simulink model "hopeForSarah"  (R2019a)
settings: Solver=ode1  StartTime=0.0  StopTime=2.5  FixedStep=Ts_Power  RelTol=1e-3
PostLoadFcn:
  | %% Init for wind PnO models - global system parameters
  | OVERRIDE_SSN_MEMORY_LIMIT=1;
  | Ts=50e-6;
  | % Ts=50e-10;
  | Ts_Power=Ts;
  | Ts_Control=2*Ts;
  | freq = 50;
  | Fnom=freq;
  | Vac=400e3;
InitFcn:
  | %% Init for wind PnO models - global system parameters
  | OVERRIDE_SSN_MEMORY_LIMIT=1;
  | Ts=50e-6;
  | % Ts=50e-10;
  | Ts_Power=Ts;
  | Ts_Control=2*Ts;
  | freq = 50;
  | Fnom=freq;
  | Vac=225e3;
values from neighbouring files (symbols this model uses):
  sub_posCap = 0.16e-006    (= 1.6e-07)    [variable.m]
  sub_posInd = 0.001400563    [variable.m]
  sub_posR = 0.036    [variable.m]
  sub_zeroCap = 0.053333e-006    (= 5.3333e-08)    [variable.m]
  sub_zeroInd = 0.00420169    [variable.m]
  sub_zeroR = 0.108    [variable.m]
  transfo_L1 = 0.05999374    [variable.m]
  transfo_L2 = 0.05999374    [variable.m]
  transfo_R1 = 0.000866667    [variable.m]
  transfo_R2 = 0.00086667    [variable.m]
undefined symbols (not defined in the file or in its folder): D1, D11, Delta, den, DiscIntNeverNeededParam, dx, find_system, gcbh, num, out_Buses, out_WindFarms, sps_rtmsupport
libraries: powerlib x284, simulink x144, powerlib_meascontrol x144, eeSinusoidalMeasurement x74, elements x52, spsVIMeasurementModel x48, simulink_extras x48, eePowerMeasurement x23
(part 3 of 30)

== system hopeForSarah/SC_Console/Subsystem ==
  In1 : Inport
  Bus Selector : BusSelector  OutputSignals=Vabc_grid (pu),Iabc_conv (pu),P_grid,Q_grid
  Bus Selector1 : BusSelector  OutputSignals=Q_grid (y: nom; b: measured),V_dc (y: nom; b: measured),I_abc (A),id,iq,theta_PLL
  Bus Selector2 : BusSelector  OutputSignals=Idc_gen+grid,I_cap+chopper,Pgrid,vdc
  Bus Selector3 : BusSelector  OutputSignals=Vabc (kV),Iabc,PQ,Pelec (MW)
  Bus Selector4 : BusSelector  OutputSignals=Vabc_pu_mag,Iabc_pu_mag,PQ,Pelec_pu
  Bus Selector5 : BusSelector  OutputSignals=WindTurbine_GridSide,WindTurbine_ConverterSide,WindTurbine_DCSide,WindTurbine_PhasetoGroundMeasurements,WindTurbine_puMeasurements,Windturbine_FaultvsGridFRTRequirements,WindTurbine_Displays
  Bus Selector6 : BusSelector  OutputSignals=Vabc pu mag,Grid Code FRT requirements
  Bus Selector7 : BusSelector  OutputSignals=Disconnection_Trigger,Time under FRT,Minimum Voltage pu,Peak POC Current pu,FRT Disconnection Time
  Bus Selector8 : BusSelector  OutputSignals=P_pu,Q_pu
  Bus Selector9 : BusSelector  OutputSignals=P (MW),Q (MVA)
  Goto14 : Goto  Commented=on  GotoTag=Pgrid  TagVisibility=global
  Goto20 : Goto  Commented=on  GotoTag=Vabc_pu_mag  TagVisibility=global
  Mux : Mux  Inputs=2
  Mux1 : Mux  Inputs=2
  tag scope: Disconnection_trigger=global, FRT_disconnection_time=global, FRT_grid_code_requirements=global, FRT_time=global, I_capANDchopper=global, Iabc=global, Iabc_conv_pu=global, Iabc_pu_mag=global, Iabc_ref=global, Idc_genANDgrid=global, Minimum_Voltage_pu=global, PQ=global, PQ_pu=global, Peak_POC_current_pu=global, Pelec=global, Pelec_pu=global, Pgrid=global, Qgrid=global, Qgrid_nomandmeas=global, Theta_PLL=global, Vabc_grid_pu=global, Vabc_kV=global, Vabc_pu_mag=global, Vdc=global, Vdc_nomandmeas=global, id=global, iq=global
  wires:
  In1/1 -> Bus Selector5/1
  Bus Selector5/1 -> Bus Selector/1  "<WindTurbine_GridSide>"
  Bus Selector5/2 -> Bus Selector1/1  "<WindTurbine_ConverterSide>"
  Bus Selector5/3 -> Bus Selector2/1  "<WindTurbine_DCSide>"
  Bus Selector5/4 -> Bus Selector3/1  "<WindTurbine_PhasetoGroundMeasurements>"
  Bus Selector5/5 -> Bus Selector4/1  "<WindTurbine_puMeasurements>"
  Bus Selector5/6 -> Bus Selector6/1  "<Windturbine_FaultvsGridFRTRequirements>"
  Bus Selector5/7 -> Bus Selector7/1  "<WindTurbine_Displays>"
  Bus Selector/1 -> [Vabc_grid_pu]  "<Vabc_grid (pu)>"
  Bus Selector/2 -> [Iabc_conv_pu]  "<Iabc_conv (pu)>"
  Bus Selector/3 -> [Pgrid]  "<P_grid>"
  Bus Selector/4 -> [Qgrid]  "<Q_grid>"
  Bus Selector1/1 -> [Qgrid_nomandmeas]  "<Q_grid (y: nom; b: measured)>"
  Bus Selector1/2 -> [Vdc_nomandmeas]  "<V_dc (y: nom; b: measured)>"
  Bus Selector1/3 -> [Iabc_ref]  "<I_abc (A)>"
  Bus Selector1/4 -> [id]  "<id>"
  Bus Selector1/5 -> [iq]  "<iq>"
  Bus Selector1/6 -> [Theta_PLL]  "<theta_PLL>"
  Bus Selector2/1 -> [Idc_genANDgrid]  "<Idc_gen+grid>"
  Bus Selector2/2 -> [I_capANDchopper]  "<I_cap+chopper>"
  Bus Selector2/3 -> Goto14/1  "<Pgrid>"
  Bus Selector2/4 -> [Vdc]  "<vdc>"
  Bus Selector3/1 -> [Vabc_kV]  "<Vabc (kV)>"
  Bus Selector3/2 -> [Iabc]  "<Iabc>"
  Bus Selector3/4 -> [Pelec]  "<Pelec (MW)>"
  Bus Selector4/1 -> [Vabc_pu_mag]  "<Vabc_pu_mag>"
  Bus Selector4/2 -> [Iabc_pu_mag]  "<Iabc_pu_mag>"
  Bus Selector4/3 -> Bus Selector8/1  "<PQ>"
  Bus Selector4/4 -> [Pelec_pu]  "<Pelec_pu>"
  Bus Selector6/1 -> Goto20/1  "<Vabc pu mag>"
  Bus Selector6/2 -> [FRT_grid_code_requirements]  "<Grid Code FRT requirements>"
  Bus Selector7/1 -> [Disconnection_trigger]  "<Disconnection_Trigger>"
  Bus Selector7/2 -> [FRT_time]  "<Time under FRT>"
  Bus Selector7/3 -> [Minimum_Voltage_pu]  "<Minimum Voltage pu>"
  Bus Selector7/4 -> [Peak_POC_current_pu]  "<Peak POC Current pu>"
  Bus Selector7/5 -> [FRT_disconnection_time]  "<FRT Disconnection Time>"
  Bus Selector8/1 -> Mux/1  "<P_pu>"
  Bus Selector8/2 -> Mux/2  "<Q_pu>"
  Mux/1 -> [PQ_pu]  "PQ (1:P_pu;2:Q_pu)"
  Mux1/1 -> [PQ]  "PQ (1:P;2:Q)"
  Bus Selector9/2 -> Mux1/2  "<Q (MVA)>"
  Bus Selector9/1 -> Mux1/1  "<P (MW)>"
  Bus Selector3/3 -> Bus Selector9/1  "<PQ>"

== system hopeForSarah/SC_Console/Subsystem1 ==
  In1 : Inport
  Bus Selector1 : BusSelector  OutputSignals=Vabc,Iabc,V mag,I mag,PQ
  tag scope: Bus_Iabc=global, Bus_Imag=global, Bus_PQ=global, Bus_Vabc=global, Bus_Vmag=global
  wires:
  In1/1 -> Bus Selector1/1
  Bus Selector1/1 -> [Bus_Vabc]  "<Vabc>"
  Bus Selector1/2 -> [Bus_Iabc]  "<Iabc>"
  Bus Selector1/5 -> [Bus_PQ]  "<PQ>"
  Bus Selector1/4 -> [Bus_Imag]  "<I mag>"
  Bus Selector1/3 -> [Bus_Vmag]  "<V mag>"

== system hopeForSarah/SC_Console/Subsystem3 ==
  Disconnection_Trigger : Inport
  String Constant1 : StringConstant  String="\"FRT limit surpassed\""
  String Constant2 : StringConstant  String="\"\""
  Switch1 : Switch  Criteria=u2 > Threshold
  Disconnection message : Outport  VectorParamsAs1DForOutWhenUnconnected=on
  wires:
  String Constant1/1 -> Switch1/1
  Switch1/1 -> Disconnection message/1  "Disconnection message"
  Disconnection_Trigger/1 -> Switch1/2
  String Constant2/1 -> Switch1/3

== system hopeForSarah/SC_Console/Subsystem4 ==
  Fault Current abc : Inport
  From A to kA : Gain  Gain=1/1000
  "Sinusoidal Measurement (PLL, Three-Phase)6" : eeSinusoidalMeasurement/Sinusoidal Measurement (PLL, Three-Phase)  Kp_LF=200  Ki_LF=2000  F0=freq  Theta0=0  Ts=-1
      settings: SourceProductBaseCode=PS
  Terminator13 : Terminator
  Terminator14 : Terminator
  a : Gain  Gain=1/1000
  Fault Current mag (kA) : Outport  VectorParamsAs1DForOutWhenUnconnected=on
  Fault Current abc (kA) : Outport  Port=2  VectorParamsAs1DForOutWhenUnconnected=on
  wires:
  From A to kA/1 -> Fault Current abc (kA)/1  "Fault Current abc (kA)"
  "Sinusoidal Measurement (PLL, Three-Phase)6"/1 -> Terminator13/1
  Fault Current abc/1 -> "Sinusoidal Measurement (PLL, Three-Phase)6"/1, From A to kA/1
  "Sinusoidal Measurement (PLL, Three-Phase)6"/2 -> Terminator14/1
  a/1 -> Fault Current mag (kA)/1  "Fault Current mag (kA)"
  "Sinusoidal Measurement (PLL, Three-Phase)6"/3 -> a/1  "Fault Current mag"

== system hopeForSarah/SC_Console/Visualization toolbox ==

== system hopeForSarah/SM_WT1/BusA ==
  Kv : Gain  Gain=Ki  SaturateOnIntegerOverflow=on  OutDataTypeStr=Inherit: Same as input  ParamDataTypeStr=Inherit: Same as input
  Kv1 : Gain  Gain=Kv  SaturateOnIntegerOverflow=on  OutDataTypeStr=Inherit: Same as input  ParamDataTypeStr=Inherit: Same as input
  Mode I : spsVIMeasurementModel/Complex  SystemSampleTime=-1
      settings: SourceProductBaseCode=PS
  Mode V : spsVIMeasurementModel/Complex  SystemSampleTime=-1
      settings: SourceProductBaseCode=PS
  Model : spsVIMeasurementModel/VI  SystemSampleTime=-1
      settings: SourceProductBaseCode=PS
  A : PMIOPort  Side=Left
  B : PMIOPort  Port=2  Side=Left
  C : PMIOPort  Port=3  Side=Left
  a : PMIOPort  Port=4  Side=Right
  b : PMIOPort  Port=5  Side=Right
  c : PMIOPort  Port=6  Side=Right
  Vabc : Outport  VectorParamsAs1DForOutWhenUnconnected=on
  Iabc : Outport  Port=2  VectorParamsAs1DForOutWhenUnconnected=on
  wires:
  Model/2 -> Kv/1
  Model/1 -> Kv1/1
  Kv/1 -> Mode I/1
  Kv1/1 -> Mode V/1
  Mode I/1 -> Iabc/1
  Mode V/1 -> Vabc/1
  connections:
  Model/RConn3 -- c/RConn1
  Model/RConn1 -- a/RConn1
  Model/RConn2 -- b/RConn1
  Model/LConn3 -- C/RConn1
  Model/LConn1 -- A/RConn1
  Model/LConn2 -- B/RConn1

== system hopeForSarah/SM_WT1/BusB ==
  Kv : Gain  Gain=Ki  SaturateOnIntegerOverflow=on  OutDataTypeStr=Inherit: Same as input  ParamDataTypeStr=Inherit: Same as input
  Kv1 : Gain  Gain=Kv  SaturateOnIntegerOverflow=on  OutDataTypeStr=Inherit: Same as input  ParamDataTypeStr=Inherit: Same as input
  Mode I : spsVIMeasurementModel/Complex  SystemSampleTime=-1
      settings: SourceProductBaseCode=PS
  Mode V : spsVIMeasurementModel/Complex  SystemSampleTime=-1
      settings: SourceProductBaseCode=PS
  Model : spsVIMeasurementModel/VI  SystemSampleTime=-1
      settings: SourceProductBaseCode=PS
  A : PMIOPort  Side=Left
  B : PMIOPort  Port=2  Side=Left
  C : PMIOPort  Port=3  Side=Left
  a : PMIOPort  Port=4  Side=Right
  b : PMIOPort  Port=5  Side=Right
  c : PMIOPort  Port=6  Side=Right
  Vabc : Outport  VectorParamsAs1DForOutWhenUnconnected=on
  Iabc : Outport  Port=2  VectorParamsAs1DForOutWhenUnconnected=on
  wires:
  Mode V/1 -> Vabc/1
  Mode I/1 -> Iabc/1
  Kv1/1 -> Mode V/1
  Kv/1 -> Mode I/1
  Model/1 -> Kv1/1
  Model/2 -> Kv/1
  connections:
  Model/LConn2 -- B/RConn1
  Model/LConn1 -- A/RConn1
  Model/LConn3 -- C/RConn1
  Model/RConn2 -- b/RConn1
  Model/RConn1 -- a/RConn1
  Model/RConn3 -- c/RConn1

== system hopeForSarah/SM_WT1/BusC ==
  Kv : Gain  Gain=Ki  SaturateOnIntegerOverflow=on  OutDataTypeStr=Inherit: Same as input  ParamDataTypeStr=Inherit: Same as input
  Kv1 : Gain  Gain=Kv  SaturateOnIntegerOverflow=on  OutDataTypeStr=Inherit: Same as input  ParamDataTypeStr=Inherit: Same as input
  Mode I : spsVIMeasurementModel/Complex  SystemSampleTime=-1
      settings: SourceProductBaseCode=PS
  Mode V : spsVIMeasurementModel/Complex  SystemSampleTime=-1
      settings: SourceProductBaseCode=PS
  Model : spsVIMeasurementModel/VI  SystemSampleTime=-1
      settings: SourceProductBaseCode=PS
  A : PMIOPort  Side=Left
  B : PMIOPort  Port=2  Side=Left
  C : PMIOPort  Port=3  Side=Left
  a : PMIOPort  Port=4  Side=Right
  b : PMIOPort  Port=5  Side=Right
  c : PMIOPort  Port=6  Side=Right
  Vabc : Outport  VectorParamsAs1DForOutWhenUnconnected=on
  Iabc : Outport  Port=2  VectorParamsAs1DForOutWhenUnconnected=on
  wires:
  Mode V/1 -> Vabc/1
  Mode I/1 -> Iabc/1
  Kv1/1 -> Mode V/1
  Kv/1 -> Mode I/1
  Model/1 -> Kv1/1
  Model/2 -> Kv/1
  connections:
  Model/LConn2 -- B/RConn1
  Model/LConn1 -- A/RConn1
  Model/LConn3 -- C/RConn1
  Model/RConn2 -- b/RConn1
  Model/RConn1 -- a/RConn1
  Model/RConn3 -- c/RConn1

== system hopeForSarah/SM_WT1/BusC1 ==
  Kv : Gain  Gain=Ki  SaturateOnIntegerOverflow=on  OutDataTypeStr=Inherit: Same as input  ParamDataTypeStr=Inherit: Same as input
  Kv1 : Gain  Gain=Kv  SaturateOnIntegerOverflow=on  OutDataTypeStr=Inherit: Same as input  ParamDataTypeStr=Inherit: Same as input
  Mode I : spsVIMeasurementModel/Complex  SystemSampleTime=-1
      settings: SourceProductBaseCode=PS
  Mode V : spsVIMeasurementModel/Complex  SystemSampleTime=-1
      settings: SourceProductBaseCode=PS
  Model : spsVIMeasurementModel/VI  SystemSampleTime=-1
      settings: SourceProductBaseCode=PS
  A : PMIOPort  Side=Left
  B : PMIOPort  Port=2  Side=Left
  C : PMIOPort  Port=3  Side=Left
  a : PMIOPort  Port=4  Side=Right
  b : PMIOPort  Port=5  Side=Right
  c : PMIOPort  Port=6  Side=Right
  Vabc : Outport  VectorParamsAs1DForOutWhenUnconnected=on
  Iabc : Outport  Port=2  VectorParamsAs1DForOutWhenUnconnected=on
  wires:
  Model/2 -> Kv/1
  Model/1 -> Kv1/1
  Kv/1 -> Mode I/1
  Kv1/1 -> Mode V/1
  Mode I/1 -> Iabc/1
  Mode V/1 -> Vabc/1
  connections:
  Model/RConn3 -- c/RConn1
  Model/RConn1 -- a/RConn1
  Model/RConn2 -- b/RConn1
  Model/LConn3 -- C/RConn1
  Model/LConn1 -- A/RConn1
  Model/LConn2 -- B/RConn1

== system hopeForSarah/SM_WT1/BusC10 ==
  Kv : Gain  Gain=Ki  SaturateOnIntegerOverflow=on  OutDataTypeStr=Inherit: Same as input  ParamDataTypeStr=Inherit: Same as input
  Kv1 : Gain  Gain=Kv  SaturateOnIntegerOverflow=on  OutDataTypeStr=Inherit: Same as input  ParamDataTypeStr=Inherit: Same as input
  Mode I : spsVIMeasurementModel/Complex  SystemSampleTime=-1
      settings: SourceProductBaseCode=PS
  Mode V : spsVIMeasurementModel/Complex  SystemSampleTime=-1
      settings: SourceProductBaseCode=PS
  Model : spsVIMeasurementModel/VI  SystemSampleTime=-1
      settings: SourceProductBaseCode=PS
  A : PMIOPort  Side=Left
  B : PMIOPort  Port=2  Side=Left
  C : PMIOPort  Port=3  Side=Left
  a : PMIOPort  Port=4  Side=Right
  b : PMIOPort  Port=5  Side=Right
  c : PMIOPort  Port=6  Side=Right
  Vabc : Outport  VectorParamsAs1DForOutWhenUnconnected=on
  Iabc : Outport  Port=2  VectorParamsAs1DForOutWhenUnconnected=on
  wires:
  Mode V/1 -> Vabc/1
  Mode I/1 -> Iabc/1
  Kv1/1 -> Mode V/1
  Kv/1 -> Mode I/1
  Model/1 -> Kv1/1
  Model/2 -> Kv/1
  connections:
  Model/LConn2 -- B/RConn1
  Model/LConn1 -- A/RConn1
  Model/LConn3 -- C/RConn1
  Model/RConn2 -- b/RConn1
  Model/RConn1 -- a/RConn1
  Model/RConn3 -- c/RConn1

== system hopeForSarah/SM_WT1/BusC11 ==
  Kv : Gain  Gain=Ki  SaturateOnIntegerOverflow=on  OutDataTypeStr=Inherit: Same as input  ParamDataTypeStr=Inherit: Same as input
  Kv1 : Gain  Gain=Kv  SaturateOnIntegerOverflow=on  OutDataTypeStr=Inherit: Same as input  ParamDataTypeStr=Inherit: Same as input
  Mode I : spsVIMeasurementModel/Complex  SystemSampleTime=-1
      settings: SourceProductBaseCode=PS
  Mode V : spsVIMeasurementModel/Complex  SystemSampleTime=-1
      settings: SourceProductBaseCode=PS
  Model : spsVIMeasurementModel/VI  SystemSampleTime=-1
      settings: SourceProductBaseCode=PS
  A : PMIOPort  Side=Left
  B : PMIOPort  Port=2  Side=Left
  C : PMIOPort  Port=3  Side=Left
  a : PMIOPort  Port=4  Side=Right
  b : PMIOPort  Port=5  Side=Right
  c : PMIOPort  Port=6  Side=Right
  Vabc : Outport  VectorParamsAs1DForOutWhenUnconnected=on
  Iabc : Outport  Port=2  VectorParamsAs1DForOutWhenUnconnected=on
  wires:
  Mode V/1 -> Vabc/1
  Mode I/1 -> Iabc/1
  Kv1/1 -> Mode V/1
  Kv/1 -> Mode I/1
  Model/1 -> Kv1/1
  Model/2 -> Kv/1
  connections:
  Model/LConn2 -- B/RConn1
  Model/LConn1 -- A/RConn1
  Model/LConn3 -- C/RConn1
  Model/RConn2 -- b/RConn1
  Model/RConn1 -- a/RConn1
  Model/RConn3 -- c/RConn1

== system hopeForSarah/SM_WT1/BusC12 ==
  Kv : Gain  Gain=Ki  SaturateOnIntegerOverflow=on  OutDataTypeStr=Inherit: Same as input  ParamDataTypeStr=Inherit: Same as input
  Kv1 : Gain  Gain=Kv  SaturateOnIntegerOverflow=on  OutDataTypeStr=Inherit: Same as input  ParamDataTypeStr=Inherit: Same as input
  Mode I : spsVIMeasurementModel/Complex  SystemSampleTime=-1
      settings: SourceProductBaseCode=PS
  Mode V : spsVIMeasurementModel/Complex  SystemSampleTime=-1
      settings: SourceProductBaseCode=PS
  Model : spsVIMeasurementModel/VI  SystemSampleTime=-1
      settings: SourceProductBaseCode=PS
  A : PMIOPort  Side=Left
  B : PMIOPort  Port=2  Side=Left
  C : PMIOPort  Port=3  Side=Left
  a : PMIOPort  Port=4  Side=Right
  b : PMIOPort  Port=5  Side=Right
  c : PMIOPort  Port=6  Side=Right
  Vabc : Outport  VectorParamsAs1DForOutWhenUnconnected=on
  Iabc : Outport  Port=2  VectorParamsAs1DForOutWhenUnconnected=on
  wires:
  Mode V/1 -> Vabc/1
  Mode I/1 -> Iabc/1
  Kv1/1 -> Mode V/1
  Kv/1 -> Mode I/1
  Model/1 -> Kv1/1
  Model/2 -> Kv/1
  connections:
  Model/LConn2 -- B/RConn1
  Model/LConn1 -- A/RConn1
  Model/LConn3 -- C/RConn1
  Model/RConn2 -- b/RConn1
  Model/RConn1 -- a/RConn1
  Model/RConn3 -- c/RConn1

== system hopeForSarah/SM_WT1/BusC2 ==
  Kv : Gain  Gain=Ki  SaturateOnIntegerOverflow=on  OutDataTypeStr=Inherit: Same as input  ParamDataTypeStr=Inherit: Same as input
  Kv1 : Gain  Gain=Kv  SaturateOnIntegerOverflow=on  OutDataTypeStr=Inherit: Same as input  ParamDataTypeStr=Inherit: Same as input
  Mode I : spsVIMeasurementModel/Complex  SystemSampleTime=-1
      settings: SourceProductBaseCode=PS
  Mode V : spsVIMeasurementModel/Complex  SystemSampleTime=-1
      settings: SourceProductBaseCode=PS
  Model : spsVIMeasurementModel/VI  SystemSampleTime=-1
      settings: SourceProductBaseCode=PS
  A : PMIOPort  Side=Left
  B : PMIOPort  Port=2  Side=Left
  C : PMIOPort  Port=3  Side=Left
  a : PMIOPort  Port=4  Side=Right
  b : PMIOPort  Port=5  Side=Right
  c : PMIOPort  Port=6  Side=Right
  Vabc : Outport  VectorParamsAs1DForOutWhenUnconnected=on
  Iabc : Outport  Port=2  VectorParamsAs1DForOutWhenUnconnected=on
  wires:
  Mode V/1 -> Vabc/1
  Mode I/1 -> Iabc/1
  Kv1/1 -> Mode V/1
  Kv/1 -> Mode I/1
  Model/1 -> Kv1/1
  Model/2 -> Kv/1
  connections:
  Model/LConn2 -- B/RConn1
  Model/LConn1 -- A/RConn1
  Model/LConn3 -- C/RConn1
  Model/RConn2 -- b/RConn1
  Model/RConn1 -- a/RConn1
  Model/RConn3 -- c/RConn1

== system hopeForSarah/SM_WT1/BusC3 ==
  Kv : Gain  Gain=Ki  SaturateOnIntegerOverflow=on  OutDataTypeStr=Inherit: Same as input  ParamDataTypeStr=Inherit: Same as input
  Kv1 : Gain  Gain=Kv  SaturateOnIntegerOverflow=on  OutDataTypeStr=Inherit: Same as input  ParamDataTypeStr=Inherit: Same as input
  Mode I : spsVIMeasurementModel/Complex  SystemSampleTime=-1
      settings: SourceProductBaseCode=PS
  Mode V : spsVIMeasurementModel/Complex  SystemSampleTime=-1
      settings: SourceProductBaseCode=PS
  Model : spsVIMeasurementModel/VI  SystemSampleTime=-1
      settings: SourceProductBaseCode=PS
  A : PMIOPort  Side=Left
  B : PMIOPort  Port=2  Side=Left
  C : PMIOPort  Port=3  Side=Left
  a : PMIOPort  Port=4  Side=Right
  b : PMIOPort  Port=5  Side=Right
  c : PMIOPort  Port=6  Side=Right
  Vabc : Outport  VectorParamsAs1DForOutWhenUnconnected=on
  Iabc : Outport  Port=2  VectorParamsAs1DForOutWhenUnconnected=on
  wires:
  Mode V/1 -> Vabc/1
  Mode I/1 -> Iabc/1
  Kv1/1 -> Mode V/1
  Kv/1 -> Mode I/1
  Model/1 -> Kv1/1
  Model/2 -> Kv/1
  connections:
  Model/LConn2 -- B/RConn1
  Model/LConn1 -- A/RConn1
  Model/LConn3 -- C/RConn1
  Model/RConn2 -- b/RConn1
  Model/RConn1 -- a/RConn1
  Model/RConn3 -- c/RConn1

== system hopeForSarah/SM_WT1/BusC4 ==
  Kv : Gain  Gain=Ki  SaturateOnIntegerOverflow=on  OutDataTypeStr=Inherit: Same as input  ParamDataTypeStr=Inherit: Same as input
  Kv1 : Gain  Gain=Kv  SaturateOnIntegerOverflow=on  OutDataTypeStr=Inherit: Same as input  ParamDataTypeStr=Inherit: Same as input
  Mode I : spsVIMeasurementModel/Complex  SystemSampleTime=-1
      settings: SourceProductBaseCode=PS
  Mode V : spsVIMeasurementModel/Complex  SystemSampleTime=-1
      settings: SourceProductBaseCode=PS
  Model : spsVIMeasurementModel/VI  SystemSampleTime=-1
      settings: SourceProductBaseCode=PS
  A : PMIOPort  Side=Left
  B : PMIOPort  Port=2  Side=Left
  C : PMIOPort  Port=3  Side=Left
  a : PMIOPort  Port=4  Side=Right
  b : PMIOPort  Port=5  Side=Right
  c : PMIOPort  Port=6  Side=Right
  Vabc : Outport  VectorParamsAs1DForOutWhenUnconnected=on
  Iabc : Outport  Port=2  VectorParamsAs1DForOutWhenUnconnected=on
  wires:
  Mode V/1 -> Vabc/1
  Mode I/1 -> Iabc/1
  Kv1/1 -> Mode V/1
  Kv/1 -> Mode I/1
  Model/1 -> Kv1/1
  Model/2 -> Kv/1
  connections:
  Model/LConn2 -- B/RConn1
  Model/LConn1 -- A/RConn1
  Model/LConn3 -- C/RConn1
  Model/RConn2 -- b/RConn1
  Model/RConn1 -- a/RConn1
  Model/RConn3 -- c/RConn1

== system hopeForSarah/SM_WT1/BusC5 ==
  Kv : Gain  Gain=Ki  SaturateOnIntegerOverflow=on  OutDataTypeStr=Inherit: Same as input  ParamDataTypeStr=Inherit: Same as input
  Kv1 : Gain  Gain=Kv  SaturateOnIntegerOverflow=on  OutDataTypeStr=Inherit: Same as input  ParamDataTypeStr=Inherit: Same as input
  Mode I : spsVIMeasurementModel/Complex  SystemSampleTime=-1
      settings: SourceProductBaseCode=PS
  Mode V : spsVIMeasurementModel/Complex  SystemSampleTime=-1
      settings: SourceProductBaseCode=PS
  Model : spsVIMeasurementModel/VI  SystemSampleTime=-1
      settings: SourceProductBaseCode=PS
  A : PMIOPort  Side=Left
  B : PMIOPort  Port=2  Side=Left
  C : PMIOPort  Port=3  Side=Left
  a : PMIOPort  Port=4  Side=Right
  b : PMIOPort  Port=5  Side=Right
  c : PMIOPort  Port=6  Side=Right
  Vabc : Outport  VectorParamsAs1DForOutWhenUnconnected=on
  Iabc : Outport  Port=2  VectorParamsAs1DForOutWhenUnconnected=on
  wires:
  Mode V/1 -> Vabc/1
  Mode I/1 -> Iabc/1
  Kv1/1 -> Mode V/1
  Kv/1 -> Mode I/1
  Model/1 -> Kv1/1
  Model/2 -> Kv/1
  connections:
  Model/LConn2 -- B/RConn1
  Model/LConn1 -- A/RConn1
  Model/LConn3 -- C/RConn1
  Model/RConn2 -- b/RConn1
  Model/RConn1 -- a/RConn1
  Model/RConn3 -- c/RConn1

== system hopeForSarah/SM_WT1/BusC6 ==
  Kv : Gain  Gain=Ki  SaturateOnIntegerOverflow=on  OutDataTypeStr=Inherit: Same as input  ParamDataTypeStr=Inherit: Same as input
  Kv1 : Gain  Gain=Kv  SaturateOnIntegerOverflow=on  OutDataTypeStr=Inherit: Same as input  ParamDataTypeStr=Inherit: Same as input
  Mode I : spsVIMeasurementModel/Complex  SystemSampleTime=-1
      settings: SourceProductBaseCode=PS
  Mode V : spsVIMeasurementModel/Complex  SystemSampleTime=-1
      settings: SourceProductBaseCode=PS
  Model : spsVIMeasurementModel/VI  SystemSampleTime=-1
      settings: SourceProductBaseCode=PS
  A : PMIOPort  Side=Left
  B : PMIOPort  Port=2  Side=Left
  C : PMIOPort  Port=3  Side=Left
  a : PMIOPort  Port=4  Side=Right
  b : PMIOPort  Port=5  Side=Right
  c : PMIOPort  Port=6  Side=Right
  Vabc : Outport  VectorParamsAs1DForOutWhenUnconnected=on
  Iabc : Outport  Port=2  VectorParamsAs1DForOutWhenUnconnected=on
  wires:
  Mode V/1 -> Vabc/1
  Mode I/1 -> Iabc/1
  Kv1/1 -> Mode V/1
  Kv/1 -> Mode I/1
  Model/1 -> Kv1/1
  Model/2 -> Kv/1
  connections:
  Model/LConn2 -- B/RConn1
  Model/LConn1 -- A/RConn1
  Model/LConn3 -- C/RConn1
  Model/RConn2 -- b/RConn1
  Model/RConn1 -- a/RConn1
  Model/RConn3 -- c/RConn1

== system hopeForSarah/SM_WT1/BusC7 ==
  Kv : Gain  Gain=Ki  SaturateOnIntegerOverflow=on  OutDataTypeStr=Inherit: Same as input  ParamDataTypeStr=Inherit: Same as input
  Kv1 : Gain  Gain=Kv  SaturateOnIntegerOverflow=on  OutDataTypeStr=Inherit: Same as input  ParamDataTypeStr=Inherit: Same as input
  Mode I : spsVIMeasurementModel/Complex  SystemSampleTime=-1
      settings: SourceProductBaseCode=PS
  Mode V : spsVIMeasurementModel/Complex  SystemSampleTime=-1
      settings: SourceProductBaseCode=PS
  Model : spsVIMeasurementModel/VI  SystemSampleTime=-1
      settings: SourceProductBaseCode=PS
  A : PMIOPort  Side=Left
  B : PMIOPort  Port=2  Side=Left
  C : PMIOPort  Port=3  Side=Left
  a : PMIOPort  Port=4  Side=Right
  b : PMIOPort  Port=5  Side=Right
  c : PMIOPort  Port=6  Side=Right
  Vabc : Outport  VectorParamsAs1DForOutWhenUnconnected=on
  Iabc : Outport  Port=2  VectorParamsAs1DForOutWhenUnconnected=on
  wires:
  Mode V/1 -> Vabc/1
  Mode I/1 -> Iabc/1
  Kv1/1 -> Mode V/1
  Kv/1 -> Mode I/1
  Model/1 -> Kv1/1
  Model/2 -> Kv/1
  connections:
  Model/LConn2 -- B/RConn1
  Model/LConn1 -- A/RConn1
  Model/LConn3 -- C/RConn1
  Model/RConn2 -- b/RConn1
  Model/RConn1 -- a/RConn1
  Model/RConn3 -- c/RConn1

== system hopeForSarah/SM_WT1/BusC8 ==
  Kv : Gain  Gain=Ki  SaturateOnIntegerOverflow=on  OutDataTypeStr=Inherit: Same as input  ParamDataTypeStr=Inherit: Same as input
  Kv1 : Gain  Gain=Kv  SaturateOnIntegerOverflow=on  OutDataTypeStr=Inherit: Same as input  ParamDataTypeStr=Inherit: Same as input
  Mode I : spsVIMeasurementModel/Complex  SystemSampleTime=-1
      settings: SourceProductBaseCode=PS
  Mode V : spsVIMeasurementModel/Complex  SystemSampleTime=-1
      settings: SourceProductBaseCode=PS
  Model : spsVIMeasurementModel/VI  SystemSampleTime=-1
      settings: SourceProductBaseCode=PS
  A : PMIOPort  Side=Left
  B : PMIOPort  Port=2  Side=Left
  C : PMIOPort  Port=3  Side=Left
  a : PMIOPort  Port=4  Side=Right
  b : PMIOPort  Port=5  Side=Right
  c : PMIOPort  Port=6  Side=Right
  Vabc : Outport  VectorParamsAs1DForOutWhenUnconnected=on
  Iabc : Outport  Port=2  VectorParamsAs1DForOutWhenUnconnected=on
  wires:
  Mode V/1 -> Vabc/1
  Mode I/1 -> Iabc/1
  Kv1/1 -> Mode V/1
  Kv/1 -> Mode I/1
  Model/1 -> Kv1/1
  Model/2 -> Kv/1
  connections:
  Model/LConn2 -- B/RConn1
  Model/LConn1 -- A/RConn1
  Model/LConn3 -- C/RConn1
  Model/RConn2 -- b/RConn1
  Model/RConn1 -- a/RConn1
  Model/RConn3 -- c/RConn1

== system hopeForSarah/SM_WT1/BusC9 ==
  Kv : Gain  Gain=Ki  SaturateOnIntegerOverflow=on  OutDataTypeStr=Inherit: Same as input  ParamDataTypeStr=Inherit: Same as input
  Kv1 : Gain  Gain=Kv  SaturateOnIntegerOverflow=on  OutDataTypeStr=Inherit: Same as input  ParamDataTypeStr=Inherit: Same as input
  Mode I : spsVIMeasurementModel/Complex  SystemSampleTime=-1
      settings: SourceProductBaseCode=PS
  Mode V : spsVIMeasurementModel/Complex  SystemSampleTime=-1
      settings: SourceProductBaseCode=PS
  Model : spsVIMeasurementModel/VI  SystemSampleTime=-1
      settings: SourceProductBaseCode=PS
  A : PMIOPort  Side=Left
  B : PMIOPort  Port=2  Side=Left
  C : PMIOPort  Port=3  Side=Left
  a : PMIOPort  Port=4  Side=Right
  b : PMIOPort  Port=5  Side=Right
  c : PMIOPort  Port=6  Side=Right
  Vabc : Outport  VectorParamsAs1DForOutWhenUnconnected=on
  Iabc : Outport  Port=2  VectorParamsAs1DForOutWhenUnconnected=on
  wires:
  Mode V/1 -> Vabc/1
  Mode I/1 -> Iabc/1
  Kv1/1 -> Mode V/1
  Kv/1 -> Mode I/1
  Model/1 -> Kv1/1
  Model/2 -> Kv/1
  connections:
  Model/LConn2 -- B/RConn1
  Model/LConn1 -- A/RConn1
  Model/LConn3 -- C/RConn1
  Model/RConn2 -- b/RConn1
  Model/RConn1 -- a/RConn1
  Model/RConn3 -- c/RConn1

== system hopeForSarah/SM_WT1/BusD ==
  Kv : Gain  Gain=Ki  SaturateOnIntegerOverflow=on  OutDataTypeStr=Inherit: Same as input  ParamDataTypeStr=Inherit: Same as input
  Kv1 : Gain  Gain=Kv  SaturateOnIntegerOverflow=on  OutDataTypeStr=Inherit: Same as input  ParamDataTypeStr=Inherit: Same as input
  Mode I : spsVIMeasurementModel/Complex  SystemSampleTime=-1
      settings: SourceProductBaseCode=PS
  Mode V : spsVIMeasurementModel/Complex  SystemSampleTime=-1
      settings: SourceProductBaseCode=PS
  Model : spsVIMeasurementModel/VI  SystemSampleTime=-1
      settings: SourceProductBaseCode=PS
  A : PMIOPort  Side=Left
  B : PMIOPort  Port=2  Side=Left
  C : PMIOPort  Port=3  Side=Left
  a : PMIOPort  Port=4  Side=Right
  b : PMIOPort  Port=5  Side=Right
  c : PMIOPort  Port=6  Side=Right
  Vabc : Outport  VectorParamsAs1DForOutWhenUnconnected=on
  Iabc : Outport  Port=2  VectorParamsAs1DForOutWhenUnconnected=on
  wires:
  Model/2 -> Kv/1
  Model/1 -> Kv1/1
  Kv/1 -> Mode I/1
  Kv1/1 -> Mode V/1
  Mode I/1 -> Iabc/1
  Mode V/1 -> Vabc/1
  connections:
  Model/RConn3 -- c/RConn1
  Model/RConn1 -- a/RConn1
  Model/RConn2 -- b/RConn1
  Model/LConn3 -- C/RConn1
  Model/LConn1 -- A/RConn1
  Model/LConn2 -- B/RConn1

== system hopeForSarah/SM_WT1/Controllable Fault ==
  Fault Base and ramp restitution V source : powerlib/Electrical Sources/Three-Phase Programmable Voltage Source  PositiveSequence="[Vac*Fault_Base_Voltage_pu  0 freq]"  VariationEntity=Amplitude  VariationType=Ramp  VariationTypeAlt=Step  VariationStep=0.5  VariationRate=Fault_Ramp_Rate_VoltageSourceBlock  VariationMagnitude=0.3  VariationFrequency=2  VariationTiming=[Fault_Start_Time+Fault_Base_Duration_time Fault_Ramp_End_Time]  VariationPhaseA=off  Amplitudes=[1 0.8 1.2 1.0]  TimeValues=[0 0.1 0.15 0.2]  HarmonicGeneration=off  HarmonicA=[3 0.2 -25 0]  HarmonicB=[2 0.15 35 2]  Timing="[0.05  3]"  BusType=swing  Pref=0  Qref=0  Qmin=-inf  Qmax=inf
  Ground3 : powerlib/Elements/Ground  LConnTagsString=a
  Three-Phase Breaker 2 : powerlib/Elements/Three-Phase Breaker  InitialState=open  SwitchA=on  SwitchB=on  SwitchC=on  SwitchTimes=[Fault_Start_Time Fault_Ramp_End_Time]  External=off  BreakerResistance=0.01  SnubberResistance=1e6  SnubberCapacitance=inf  Measurements=None
  A : PMIOPort  Side=Right
  B : PMIOPort  Port=2  Side=Right
  C : PMIOPort  Port=3  Side=Right
  connections:
  C/RConn1 -- Three-Phase Breaker 2/RConn3
  Three-Phase Breaker 2/RConn1 -- A/RConn1
  Fault Base and ramp restitution V source/LConn1 -- Ground3/LConn1
  Three-Phase Breaker 2/RConn2 -- B/RConn1
  Three-Phase Breaker 2/LConn1 -- Fault Base and ramp restitution V source/RConn1
  Three-Phase Breaker 2/LConn3 -- Fault Base and ramp restitution V source/RConn3
  Three-Phase Breaker 2/LConn2 -- Fault Base and ramp restitution V source/RConn2

== system hopeForSarah/SM_WT1/Differential Element 1 ==
  Iabc Remote : Inport
  Iabc Local : Inport  Port=2
  Vabc Local : Inport  Port=3
  Enable : EnablePort
  *1 : Gain  Gain=CT_local*CT_local_dir  SaturateOnIntegerOverflow=on  OutDataTypeStr=Inherit: Same as input  ParamDataTypeStr=Inherit: Same as input
  *2 : Gain  Gain=CT_local*CT_local_dir  SaturateOnIntegerOverflow=on  OutDataTypeStr=Inherit: Same as input  ParamDataTypeStr=Inherit: Same as input
  *3 : Gain  Gain=CT_local*CT_local_dir  SaturateOnIntegerOverflow=on  OutDataTypeStr=Inherit: Same as input  ParamDataTypeStr=Inherit: Same as input
  *4 : Gain  Gain=PT_local  SaturateOnIntegerOverflow=on  OutDataTypeStr=Inherit: Same as input  ParamDataTypeStr=Inherit: Same as input
  *5 : Gain  Gain=PT_local  SaturateOnIntegerOverflow=on  OutDataTypeStr=Inherit: Same as input  ParamDataTypeStr=Inherit: Same as input
  *6 : Gain  Gain=PT_local  SaturateOnIntegerOverflow=on  OutDataTypeStr=Inherit: Same as input  ParamDataTypeStr=Inherit: Same as input
  *7 : Gain  Gain=CT_remote*CT_remote_dir  SaturateOnIntegerOverflow=on  OutDataTypeStr=Inherit: Same as input  ParamDataTypeStr=Inherit: Same as input
  *8 : Gain  Gain=CT_remote*CT_remote_dir  SaturateOnIntegerOverflow=on  OutDataTypeStr=Inherit: Same as input  ParamDataTypeStr=Inherit: Same as input
  *9 : Gain  Gain=CT_remote*CT_remote_dir  SaturateOnIntegerOverflow=on  OutDataTypeStr=Inherit: Same as input  ParamDataTypeStr=Inherit: Same as input
  Data Type Conversion : DataTypeConversion  OutDataTypeStr=boolean
  Data Type Conversion1 : DataTypeConversion  OutDataTypeStr=boolean
  Data Type Conversion2 : DataTypeConversion  OutDataTypeStr=boolean
  Demux1 : Demux  Outputs=3
  Demux2 : Demux  Outputs=3
  Demux3 : Demux  Outputs=3
  Main Protection (Current Differential) : Subsystem
  Trip1 : Logic  Operator=OR  Inputs=3
  Trip : Outport  VectorParamsAs1DForOutWhenUnconnected=on
  wires:
  *9/1 -> Main Protection (Current Differential)/9(ICR)
  *8/1 -> Main Protection (Current Differential)/8(IBR)
  *7/1 -> Main Protection (Current Differential)/7(IAR)
  *6/1 -> Main Protection (Current Differential)/6(VC)
  *5/1 -> Main Protection (Current Differential)/5(VB)
  *4/1 -> Main Protection (Current Differential)/4(VA)
  *3/1 -> Main Protection (Current Differential)/3(IC)
  *1/1 -> Main Protection (Current Differential)/2(IB)
  *2/1 -> Main Protection (Current Differential)/1(IA)
  Data Type Conversion/1 -> Trip1/1
  Data Type Conversion2/1 -> Trip1/3
  Data Type Conversion1/1 -> Trip1/2
  Demux1/3 -> *6/1
  Demux1/2 -> *5/1
  Demux1/1 -> *4/1
  Demux2/3 -> *3/1
  Demux2/2 -> *1/1
  Demux2/1 -> *2/1
  Demux3/3 -> *9/1
  Demux3/2 -> *8/1
  Demux3/1 -> *7/1
  Main Protection (Current Differential)/3(Trip C) -> Data Type Conversion2/1
  Main Protection (Current Differential)/2(Trip B) -> Data Type Conversion1/1
  Main Protection (Current Differential)/1(Trip A) -> Data Type Conversion/1
  Trip1/1 -> Trip/1
  Iabc Remote/1 -> Demux3/1
  Iabc Local/1 -> Demux2/1
  Vabc Local/1 -> Demux1/1

== system hopeForSarah/SM_WT1/Differential Element 2 ==
  Iabc Remote : Inport
  Iabc Local : Inport  Port=2
  Vabc Local : Inport  Port=3
  Enable : EnablePort
  *1 : Gain  Gain=CT_local*CT_local_dir  SaturateOnIntegerOverflow=on  OutDataTypeStr=Inherit: Same as input  ParamDataTypeStr=Inherit: Same as input
  *2 : Gain  Gain=CT_local*CT_local_dir  SaturateOnIntegerOverflow=on  OutDataTypeStr=Inherit: Same as input  ParamDataTypeStr=Inherit: Same as input
  *3 : Gain  Gain=CT_local*CT_local_dir  SaturateOnIntegerOverflow=on  OutDataTypeStr=Inherit: Same as input  ParamDataTypeStr=Inherit: Same as input
  *4 : Gain  Gain=PT_local  SaturateOnIntegerOverflow=on  OutDataTypeStr=Inherit: Same as input  ParamDataTypeStr=Inherit: Same as input
  *5 : Gain  Gain=PT_local  SaturateOnIntegerOverflow=on  OutDataTypeStr=Inherit: Same as input  ParamDataTypeStr=Inherit: Same as input
  *6 : Gain  Gain=PT_local  SaturateOnIntegerOverflow=on  OutDataTypeStr=Inherit: Same as input  ParamDataTypeStr=Inherit: Same as input
  *7 : Gain  Gain=CT_remote*CT_remote_dir  SaturateOnIntegerOverflow=on  OutDataTypeStr=Inherit: Same as input  ParamDataTypeStr=Inherit: Same as input
  *8 : Gain  Gain=CT_remote*CT_remote_dir  SaturateOnIntegerOverflow=on  OutDataTypeStr=Inherit: Same as input  ParamDataTypeStr=Inherit: Same as input
  *9 : Gain  Gain=CT_remote*CT_remote_dir  SaturateOnIntegerOverflow=on  OutDataTypeStr=Inherit: Same as input  ParamDataTypeStr=Inherit: Same as input
  Data Type Conversion : DataTypeConversion  OutDataTypeStr=boolean
  Data Type Conversion1 : DataTypeConversion  OutDataTypeStr=boolean
  Data Type Conversion2 : DataTypeConversion  OutDataTypeStr=boolean
  Demux1 : Demux  Outputs=3
  Demux2 : Demux  Outputs=3
  Demux3 : Demux  Outputs=3
  Main Protection (Current Differential) : Subsystem
  Trip1 : Logic  Operator=OR  Inputs=3
  Trip : Outport  VectorParamsAs1DForOutWhenUnconnected=on
  wires:
  *9/1 -> Main Protection (Current Differential)/9(ICR)
  *8/1 -> Main Protection (Current Differential)/8(IBR)
  *7/1 -> Main Protection (Current Differential)/7(IAR)
  *6/1 -> Main Protection (Current Differential)/6(VC)
  *5/1 -> Main Protection (Current Differential)/5(VB)
  *4/1 -> Main Protection (Current Differential)/4(VA)
  *3/1 -> Main Protection (Current Differential)/3(IC)
  *1/1 -> Main Protection (Current Differential)/2(IB)
  *2/1 -> Main Protection (Current Differential)/1(IA)
  Data Type Conversion/1 -> Trip1/1
  Data Type Conversion2/1 -> Trip1/3
  Data Type Conversion1/1 -> Trip1/2
  Demux1/3 -> *6/1
  Demux1/2 -> *5/1
  Demux1/1 -> *4/1
  Demux2/3 -> *3/1
  Demux2/2 -> *1/1
  Demux2/1 -> *2/1
  Demux3/3 -> *9/1
  Demux3/2 -> *8/1
  Demux3/1 -> *7/1
  Main Protection (Current Differential)/3(Trip C) -> Data Type Conversion2/1
  Main Protection (Current Differential)/2(Trip B) -> Data Type Conversion1/1
  Main Protection (Current Differential)/1(Trip A) -> Data Type Conversion/1
  Trip1/1 -> Trip/1
  Iabc Remote/1 -> Demux3/1
  Iabc Local/1 -> Demux2/1
  Vabc Local/1 -> Demux1/1

== system hopeForSarah/SM_WT1/Dummy Bus Signals  ==
  note: This subsystem creates a bus with the correct names and dimensions but with zeros throughout. This is required so that we can have the 'blank' from/goto tags connected to the signal switch.
  Bus Creator : BusCreator  Inputs=5
  Bus Creator1 : BusCreator  Inputs=2
  Constant : Constant  Value=[0 0 0]
  Constant1 : Constant  Value=[0 0 0 ]
  Constant{2..5} (4 alike) : Constant  Value=0
  Out1 : Outport  VectorParamsAs1DForOutWhenUnconnected=on
  wires:
  Constant/1 -> Bus Creator/1  "Vabc"
  Constant2/1 -> Bus Creator/3  "V mag"
  Constant3/1 -> Bus Creator/4  "I mag"
  Constant1/1 -> Bus Creator/2  "Iabc"
  Bus Creator/1 -> Out1/1
  Bus Creator1/1 -> Bus Creator/5  "PQ"
  Constant4/1 -> Bus Creator1/1  "P (MW)"
  Constant5/1 -> Bus Creator1/2  "Q (MVAr)"

== system hopeForSarah/SM_WT1/Dummy WF signals ==
  note: This subsystem creates a bus with the correct names and dimensions but with zeros throughout. This is required so that we can have the 'blank' from/goto tags connected to the signal switch.
  Bus Creator : BusCreator  Inputs=7
  Bus Creator{1..4,7} (5 alike) : BusCreator  Inputs=2
  Bus Creator10 : BusCreator  Inputs=6
  Bus Creator{5..6,9,11} (4 alike) : BusCreator  Inputs=4
  Bus Creator8 : BusCreator  Inputs=5
  Constant{,1..2,4,6..10,12..18,20..24,26..28,30..35} (30 alike) : Constant  Value=0
  Constant{3,5,11,19,29} (5 alike) : Constant  Value=[0 0 0]
  Mux2 : Mux  Inputs=2
  Mux3 : Mux  Inputs=2
  m : Outport  VectorParamsAs1DForOutWhenUnconnected=on
  wires:
  Constant10/1 -> Bus Creator9/3  "P_grid"
  Constant18/1 -> Bus Creator11/4  "vdc"
  Constant33/1 -> Bus Creator8/3  "Minimum Voltage pu"
  Constant/1 -> Mux3/1  "Qnom_grid"
  Constant7/1 -> Bus Creator10/5  "iq"
  Constant11/1 -> Bus Creator9/2  "Iabc_conv (pu)"
  Constant26/1 -> Bus Creator4/1  "P_pu"
  [Windturbine_PhasetoGroundMeasurements] -> Bus Creator/4  "WindTurbine_PhasetoGroundMeasurements"
  [WindTurbine_Displays] -> Bus Creator/7  "WindTurbine_Displays"
  [Windturbine_ConverterSide] -> Bus Creator/2  "WindTurbine_ConverterSide"
  Constant14/1 -> Bus Creator1/2  "Idc grid"
  Constant15/1 -> Bus Creator2/1  "I cap"
  Mux3/1 -> Bus Creator10/1  "Q_grid (y: nom; b: measured)"
  Constant12/1 -> Bus Creator6/1  "Vabc_pu_mag"
  Constant5/1 -> Bus Creator9/1  "Vabc_grid (pu)"
  Constant34/1 -> Bus Creator8/4  "Peak POC Current pu"
  Bus Creator11/1 -> [Windturbine_DCSide]
  Bus Creator/1 -> m/1
  Bus Creator9/1 -> [Windturbine_GridSide]
  Constant24/1 -> Bus Creator7/1  "Vabc pu mag"
  Constant30/1 -> Bus Creator7/2  "Grid Code FRT requirements"
  Constant4/1 -> Mux2/2  "Vdc"
  Constant9/1 -> Bus Creator9/4  "Q_grid"
  Bus Creator3/1 -> Bus Creator5/3  "PQ"
  Constant3/1 -> Bus Creator5/2  "Iabc"
  Constant23/1 -> Bus Creator6/2  "Iabc_pu_mag"
  Constant19/1 -> Bus Creator5/1  "Vabc (kV)"
  Constant2/1 -> Mux2/1  "Vdc_nom"
  Constant32/1 -> Bus Creator8/2  "Time under FRT"
  Constant6/1 -> Bus Creator10/4  "id"
  Bus Creator7/1 -> [Windturbine_FaultvsGridFRTRequirements]  "Windturbine_FaultvsGridFRTRequirements"
  Bus Creator5/1 -> [Windturbine_PhasetoGroundMeasurements]  "WindTurbine_PhasetoGroundMeasurements"
  [Windturbine_FaultvsGridFRTRequirements] -> Bus Creator/6  "Windturbine_FaultvsGridFRTRequirements"
  Constant20/1 -> Bus Creator3/1  "P (MW)"
  [Windturbine_GridSide] -> Bus Creator/1  "WindTurbine_GridSide"
  Constant29/1 -> Bus Creator10/3  "I_abc (A)"
  Bus Creator4/1 -> Bus Creator6/3  "PQ"
  Constant28/1 -> Bus Creator6/4  "Pelec_pu"
  [Windturbine_DCSide] -> Bus Creator/3  "WindTurbine_DCSide"
  Mux2/1 -> Bus Creator10/2  "V_dc (y: nom; b: measured)"
  Constant21/1 -> Bus Creator3/2  "Q (MVA)"
  Bus Creator2/1 -> Bus Creator11/2  "I_cap+chopper"
  Constant8/1 -> Bus Creator10/6  "theta_PLL"
  [Windturbine_puMeasurements] -> Bus Creator/5  "WindTurbine_puMeasurements"
  Constant13/1 -> Bus Creator1/1  "Idc gen"
  Constant22/1 -> Bus Creator5/4  "Pelec (MW)"
  Constant16/1 -> Bus Creator2/2  "I chopper"
  Constant1/1 -> Mux3/2  "Q_grid"
  Constant17/1 -> Bus Creator11/3  "Pgrid"
  Constant31/1 -> Bus Creator8/1  "Disconnection_Trigger"
  Bus Creator10/1 -> [Windturbine_ConverterSide]
  Constant27/1 -> Bus Creator4/2  "Q_pu"
  Bus Creator6/1 -> [Windturbine_puMeasurements]  "WindTurbine_puMeasurements"
  Constant35/1 -> Bus Creator8/5  "FRT Disconnection Time"
  Bus Creator1/1 -> Bus Creator11/1  "Idc_gen+grid"
  Bus Creator8/1 -> [WindTurbine_Displays]  "WindTurbine_Displays"

== system hopeForSarah/SM_WT1/Fault_timing_generator ==
  fault_params : Inport
  pulse : Inport  Port=2
  Bus Selector1 : BusSelector  OutputSignals=start_time,duration
  Constant : Constant  Value=10
  Data Type Conversion : DataTypeConversion  OutDataTypeStr=double
  Scope : Scope
  Scope1 : Scope
  faultgen : Subsystem
  sawtooth : Subsystem
  fault : Outport  VectorParamsAs1DForOutWhenUnconnected=on
  acqu : Outport  Port=2  VectorParamsAs1DForOutWhenUnconnected=on
  wires:
  sawtooth/1(sawtooth) -> Scope/1, faultgen/1(t)
  faultgen/1(fault) -> Scope1/1, Data Type Conversion/1  "fault signal"
  pulse/1 -> sawtooth/2(pules)  "synchronous pulse if no pulse,  must connect to positive"
  sawtooth/2(trig) -> acqu/1  "acquisition signal"
  fault_params/1 -> Bus Selector1/1
  Bus Selector1/1 -> faultgen/2(Tstat)  "<start_time>"
  Bus Selector1/2 -> faultgen/3(Tdur)  "<duration>"
  Data Type Conversion/1 -> fault/1
  Constant/1 -> sawtooth/1(Taqu)

== system hopeForSarah/SM_WT1/Impedance Element 1 ==
  Vabc : Inport
  Iabc : Inport  Port=2
  Enable : EnablePort
  Impedance Relay Scheme : Subsystem  mask{fCut=250, fSampling=freq*32, WindowSize=10, VoltageRange=110/sqrt(3), CurrentRange=40, ZoneTime=ZoneTime, ZoneImpedance=ZoneImpedance, LineAngle=LineAngle, k0m1=k0m1, k0a1=k0a1, underV=underV}
      mask prompts: fCut "fCut (Hz):"; fSampling "fSampling (Hz):"; WindowSize "Window Size (samples):"; VoltageRange "Voltage Range (V):"; CurrentRange "Current Range (A):"; ZoneTime "Zone Times:"; ZoneImpedance "Zone Impedances:"; LineAngle "Line Angle:"; underV "UnderVoltage Threshold (V):"
  Terminator : Terminator
  Terminator1 : Terminator
  Terminator2 : Terminator
  Trip : Outport  InitialOutput=0  VectorParamsAs1DForOutWhenUnconnected=on
  wires:
  Impedance Relay Scheme/1("TRIP ") -> Trip/1
  Vabc/1 -> Impedance Relay Scheme/1(Vabc)
  Iabc/1 -> Impedance Relay Scheme/2(Iabc)
  Impedance Relay Scheme/2(Logic) -> Terminator/1
  Impedance Relay Scheme/4(FaultZone) -> Terminator2/1
  Impedance Relay Scheme/3(FaultType) -> Terminator1/1

== system hopeForSarah/SM_WT1/Impedance Element 2 ==
  Vabc : Inport
  Iabc : Inport  Port=2
  Enable : EnablePort
  Impedance Relay Scheme : Subsystem  mask{fCut=250, fSampling=freq*32, WindowSize=10, VoltageRange=110/sqrt(3), CurrentRange=40, ZoneTime=ZoneTime, ZoneImpedance=ZoneImpedance, LineAngle=LineAngle, k0m1=k0m1, k0a1=k0a1, underV=underV}
      mask prompts: fCut "fCut (Hz):"; fSampling "fSampling (Hz):"; WindowSize "Window Size (samples):"; VoltageRange "Voltage Range (V):"; CurrentRange "Current Range (A):"; ZoneTime "Zone Times:"; ZoneImpedance "Zone Impedances:"; LineAngle "Line Angle:"; underV "UnderVoltage Threshold (V):"
  Terminator : Terminator
  Terminator1 : Terminator
  Terminator2 : Terminator
  Trip : Outport  InitialOutput=0  VectorParamsAs1DForOutWhenUnconnected=on
  wires:
  Impedance Relay Scheme/1("TRIP ") -> Trip/1
  Vabc/1 -> Impedance Relay Scheme/1(Vabc)
  Iabc/1 -> Impedance Relay Scheme/2(Iabc)
  Impedance Relay Scheme/2(Logic) -> Terminator/1
  Impedance Relay Scheme/4(FaultZone) -> Terminator2/1
  Impedance Relay Scheme/3(FaultType) -> Terminator1/1

== system hopeForSarah/SM_WT1/Overcurrent Element 1 ==
  Iabc : Inport
  Enable : EnablePort
  Overcurrent Relay Scheme : Subsystem  mask{fCut=250, fSampling=Freq*32, WindowSize=10, VoltageRange=110/sqrt(3), CurrentRange=40, Td=Td, Top=Iop, ResCurr=ResCurr}
      mask prompts: fCut "fCut (Hz):"; fSampling "fSampling (Hz):"; WindowSize "Window Size (samples):"; VoltageRange "Voltage Range (V):"; CurrentRange "Current Range (A):"; Td "Time Delay (s):"; Top "Pickup Current (A):"; ResCurr "Residual Current (A):"
  Terminator : Terminator
  Terminator1 : Terminator
  Trip : Outport  InitialOutput=0  VectorParamsAs1DForOutWhenUnconnected=on
  wires:
  Iabc/1 -> Overcurrent Relay Scheme/1(Iabc)
  Overcurrent Relay Scheme/1("TRIP ") -> Trip/1
  Overcurrent Relay Scheme/2(Logic) -> Terminator/1
  Overcurrent Relay Scheme/3(FaultType) -> Terminator1/1

== system hopeForSarah/SM_WT1/Overcurrent Element 2 ==
  Iabc : Inport
  Enable : EnablePort
  Overcurrent Relay Scheme : Subsystem  mask{fCut=250, fSampling=Freq*32, WindowSize=10, VoltageRange=110/sqrt(3), CurrentRange=40, Td=Td, Top=Iop, ResCurr=ResCurr}
      mask prompts: fCut "fCut (Hz):"; fSampling "fSampling (Hz):"; WindowSize "Window Size (samples):"; VoltageRange "Voltage Range (V):"; CurrentRange "Current Range (A):"; Td "Time Delay (s):"; Top "Pickup Current (A):"; ResCurr "Residual Current (A):"
  Terminator : Terminator
  Terminator1 : Terminator
  Trip : Outport  InitialOutput=0  VectorParamsAs1DForOutWhenUnconnected=on
  wires:
  Iabc/1 -> Overcurrent Relay Scheme/1(Iabc)
  Overcurrent Relay Scheme/1("TRIP ") -> Trip/1
  Overcurrent Relay Scheme/2(Logic) -> Terminator/1
  Overcurrent Relay Scheme/3(FaultType) -> Terminator1/1

== system hopeForSarah/SM_WT1/Overcurrent Inverse time ==
  Iabc : Inport
  Enable : EnablePort
  Overcurrent Relay Scheme : Subsystem  mask{fCut=250, fSampling=Freq*32, WindowSize=10, VoltageRange=110/sqrt(3), CurrentRange=40, Top=Iop}
      mask prompts: fCut "fCut (Hz):"; fSampling "fSampling (Hz):"; WindowSize "Window Size (samples):"; VoltageRange "Voltage Range (V):"; CurrentRange "Current Range (A):"; Top "Pickup Current (A):"
  Terminator1 : Terminator
  Trip : Outport  InitialOutput=0  VectorParamsAs1DForOutWhenUnconnected=on
  wires:
  Iabc/1 -> Overcurrent Relay Scheme/1(Iabc)
  Overcurrent Relay Scheme/1("TRIP ") -> Trip/1
  Overcurrent Relay Scheme/2(FaultType) -> Terminator1/1

== system hopeForSarah/SM_WT1/Subsystem1 ==
  V : Inport
  I : Inport  Port=2
  Bus Creator : BusCreator  Inputs=5
  Subsystem : Subsystem
  Out1 : Outport  VectorParamsAs1DForOutWhenUnconnected=on
  wires:
  Subsystem/1(Vabc) -> Bus Creator/1  "Vabc"
  Subsystem/3(V mag) -> Bus Creator/3  "V mag"
  V/1 -> Subsystem/1(V)
  Subsystem/4(I mag) -> Bus Creator/4  "I mag"
  Subsystem/5(PQ) -> Bus Creator/5  "PQ"
  Subsystem/2(Iabc) -> Bus Creator/2  "Iabc"
  Bus Creator/1 -> Out1/1
  I/1 -> Subsystem/2(I)

== system hopeForSarah/SM_WT1/Subsystem10 ==
  V : Inport
  I : Inport  Port=2
  Bus Creator : BusCreator  Inputs=5
  Subsystem : Subsystem
  Out1 : Outport  VectorParamsAs1DForOutWhenUnconnected=on
  wires:
  I/1 -> Subsystem/2(I)
  Bus Creator/1 -> Out1/1
  Subsystem/2(Iabc) -> Bus Creator/2  "Iabc"
  Subsystem/5(PQ) -> Bus Creator/5  "PQ"
  Subsystem/4(I mag) -> Bus Creator/4  "I mag"
  V/1 -> Subsystem/1(V)
  Subsystem/3(V mag) -> Bus Creator/3  "V mag"
  Subsystem/1(Vabc) -> Bus Creator/1  "Vabc"

== system hopeForSarah/SM_WT1/Subsystem11 ==
  V : Inport
  I : Inport  Port=2
  Bus Creator : BusCreator  Inputs=5
  Subsystem : Subsystem
  Out1 : Outport  VectorParamsAs1DForOutWhenUnconnected=on
  wires:
  I/1 -> Subsystem/2(I)
  Bus Creator/1 -> Out1/1
  Subsystem/2(Iabc) -> Bus Creator/2  "Iabc"
  Subsystem/5(PQ) -> Bus Creator/5  "PQ"
  Subsystem/4(I mag) -> Bus Creator/4  "I mag"
  V/1 -> Subsystem/1(V)
  Subsystem/3(V mag) -> Bus Creator/3  "V mag"
  Subsystem/1(Vabc) -> Bus Creator/1  "Vabc"

== system hopeForSarah/SM_WT1/Subsystem12 ==
  V : Inport
  I : Inport  Port=2
  Bus Creator : BusCreator  Inputs=5
  Subsystem : Subsystem
  Out1 : Outport  VectorParamsAs1DForOutWhenUnconnected=on
  wires:
  I/1 -> Subsystem/2(I)
  Bus Creator/1 -> Out1/1
  Subsystem/2(Iabc) -> Bus Creator/2  "Iabc"
  Subsystem/5(PQ) -> Bus Creator/5  "PQ"
  Subsystem/4(I mag) -> Bus Creator/4  "I mag"
  V/1 -> Subsystem/1(V)
  Subsystem/3(V mag) -> Bus Creator/3  "V mag"
  Subsystem/1(Vabc) -> Bus Creator/1  "Vabc"

== system hopeForSarah/SM_WT1/Subsystem13 ==
  V : Inport
  I : Inport  Port=2
  Bus Creator : BusCreator  Inputs=5
  Subsystem : Subsystem
  Out1 : Outport  VectorParamsAs1DForOutWhenUnconnected=on
  wires:
  I/1 -> Subsystem/2(I)
  Bus Creator/1 -> Out1/1
  Subsystem/2(Iabc) -> Bus Creator/2  "Iabc"
  Subsystem/5(PQ) -> Bus Creator/5  "PQ"
  Subsystem/4(I mag) -> Bus Creator/4  "I mag"
  V/1 -> Subsystem/1(V)
  Subsystem/3(V mag) -> Bus Creator/3  "V mag"
  Subsystem/1(Vabc) -> Bus Creator/1  "Vabc"

== system hopeForSarah/SM_WT1/Subsystem14 ==
  V : Inport
  I : Inport  Port=2
  Bus Creator : BusCreator  Inputs=5
  Subsystem : Subsystem
  Out1 : Outport  VectorParamsAs1DForOutWhenUnconnected=on
  wires:
  I/1 -> Subsystem/2(I)
  Bus Creator/1 -> Out1/1
  Subsystem/2(Iabc) -> Bus Creator/2  "Iabc"
  Subsystem/5(PQ) -> Bus Creator/5  "PQ"
  Subsystem/4(I mag) -> Bus Creator/4  "I mag"
  V/1 -> Subsystem/1(V)
  Subsystem/3(V mag) -> Bus Creator/3  "V mag"
  Subsystem/1(Vabc) -> Bus Creator/1  "Vabc"

== system hopeForSarah/SM_WT1/Subsystem2 ==
  V : Inport
  I : Inport  Port=2
  Bus Creator : BusCreator  Inputs=5
  Subsystem : Subsystem
  Out1 : Outport  VectorParamsAs1DForOutWhenUnconnected=on
  wires:
  I/1 -> Subsystem/2(I)
  Bus Creator/1 -> Out1/1
  Subsystem/2(Iabc) -> Bus Creator/2  "Iabc"
  Subsystem/5(PQ) -> Bus Creator/5  "PQ"
  Subsystem/4(I mag) -> Bus Creator/4  "I mag"
  V/1 -> Subsystem/1(V)
  Subsystem/3(V mag) -> Bus Creator/3  "V mag"
  Subsystem/1(Vabc) -> Bus Creator/1  "Vabc"

== system hopeForSarah/SM_WT1/Subsystem3 ==
  V : Inport
  I : Inport  Port=2
  Bus Creator : BusCreator  Inputs=5
  Subsystem : Subsystem
  Out1 : Outport  VectorParamsAs1DForOutWhenUnconnected=on
  wires:
  I/1 -> Subsystem/2(I)
  Bus Creator/1 -> Out1/1
  Subsystem/2(Iabc) -> Bus Creator/2  "Iabc"
  Subsystem/5(PQ) -> Bus Creator/5  "PQ"
  Subsystem/4(I mag) -> Bus Creator/4  "I mag"
  V/1 -> Subsystem/1(V)
  Subsystem/3(V mag) -> Bus Creator/3  "V mag"
  Subsystem/1(Vabc) -> Bus Creator/1  "Vabc"

== system hopeForSarah/SM_WT1/Subsystem4 ==
  V : Inport
  I : Inport  Port=2
  Bus Creator : BusCreator  Inputs=5
  Subsystem : Subsystem
  Out1 : Outport  VectorParamsAs1DForOutWhenUnconnected=on
  wires:
  Subsystem/1(Vabc) -> Bus Creator/1  "Vabc"
  Subsystem/3(V mag) -> Bus Creator/3  "V mag"
  V/1 -> Subsystem/1(V)
  Subsystem/4(I mag) -> Bus Creator/4  "I mag"
  Subsystem/5(PQ) -> Bus Creator/5  "PQ"
  Subsystem/2(Iabc) -> Bus Creator/2  "Iabc"
  Bus Creator/1 -> Out1/1
  I/1 -> Subsystem/2(I)
